simulink model "Prob3_MBD"  (R2020b)
settings: Solver=VariableStepAuto  StartTime=0.0  StopTime=1050  RelTol=1e-3
settings Model: Creator=Ani  LastModifiedBy=Ani
settings DataIOCC: ExternalInput=[t, noise]  LoadExternalInput=on  SaveFormat=Array

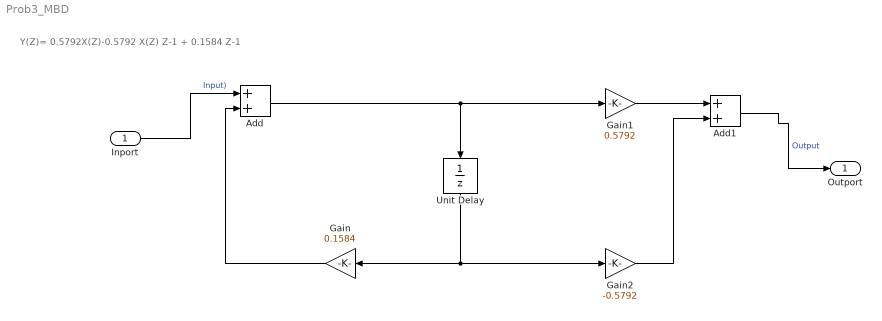
== system Prob3_MBD ==
  note: Y(Z)= 0.5792X(Z)-0.5792 X(Z) Z-1 + 0.1584 Z-1
  Inport : Inport
  Add : Sum
  Add1 : Sum
  Gain : Gain  Gain=0.1584
  Gain1 : Gain  Gain=0.5792
  Gain2 : Gain  Gain=-0.5792
  Unit Delay : UnitDelay  SampleTime=-1  HasFrameUpgradeWarning=on
  Outport : Outport
  wires:
  Gain2/1 -> Add1/2
  Add/1 -> Unit Delay/1, Gain1/1
  Add1/1 -> Outport/1  "Output"
  Inport/1 -> Add/1  "Input)"
  Unit Delay/1 -> Gain2/1, Gain/1
  Gain/1 -> Add/2
  Gain1/1 -> Add1/1
